simulink model "jointSpaceTrajController"  (Simulink 8.0)
settings: Solver=FixedStepDiscrete  StartTime=0.0  StopTime=10.0  FixedStep=Ts  RelTol=1e-3
libraries: WBCLibrary x5
settings Model: Creator=nunoguedelha  LastModifiedBy=nunoguedelha

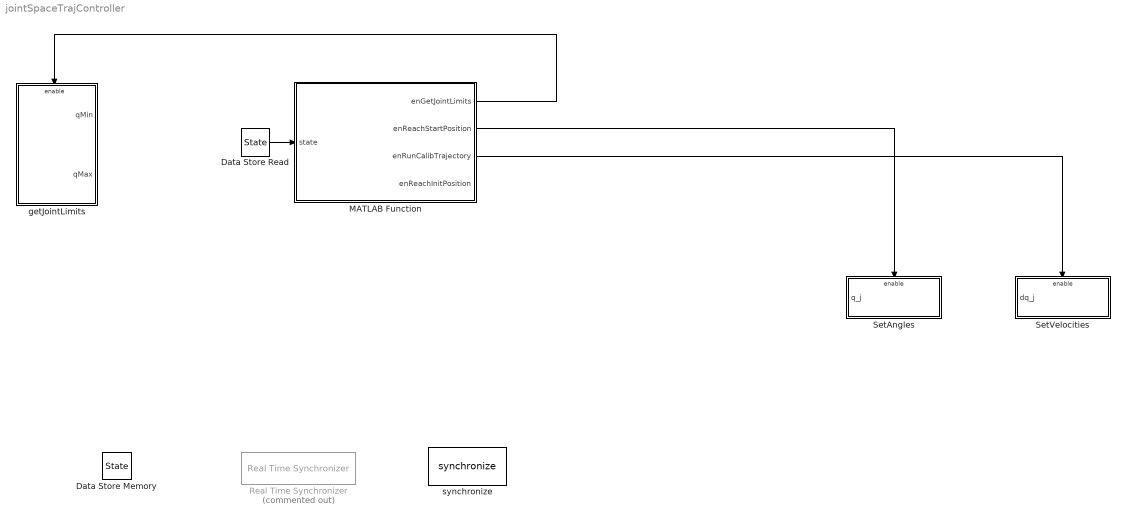
== system jointSpaceTrajController ==
  Data Store Memory : DataStoreMemory  DataStoreName=State  ReadBeforeWriteMsg=warning  WriteAfterWriteMsg=warning  WriteAfterReadMsg=warning  InitialValue=getJointLimits  OutMin=1  OutMax=4  OutDataTypeStr=Enum: SMstates
  Data Store Read : DataStoreRead  DataStoreName=State  DataStoreElements=State
  MATLAB Function : MATLAB Function  TreatAsAtomicUnit=on
  Real Time Synchronizer : WBCLibrary/Utilities/Real Time Synchronizer  Priority=-10  Commented=on  threadPeriod=Ts
  SetAngles : Subsystem  TreatAsAtomicUnit=on
  SetVelocities : Subsystem  TreatAsAtomicUnit=on
  getJointLimits : Subsystem  TreatAsAtomicUnit=on
  synchronize : WBCLibrary/Utilities/synchronize  rate=0.010  scaleFactor=1
  wires:
  MATLAB Function/2(enReachStartPosition) -> SetAngles/Enable
  MATLAB Function/3(enRunCalibTrajectory) -> SetVelocities/Enable
  MATLAB Function/1(enGetJointLimits) -> getJointLimits/Enable
  ? -> SetAngles/1(q_j)
  ? -> SetVelocities/1(dq_j)
  Data Store Read/1 -> MATLAB Function/1(state)

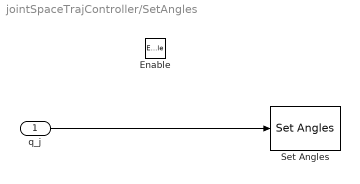
== system jointSpaceTrajController/SetAngles ==
  q_j : Inport
  Enable : EnablePort
  Set Angles : WBCLibrary/wholeBodyActuators/Set Angles  val=5  robotName=robotName  localName=localName
  wires:
  q_j/1 -> Set Angles/1

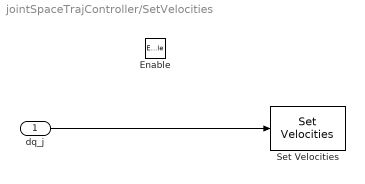
== system jointSpaceTrajController/SetVelocities ==
  dq_j : Inport
  Enable : EnablePort
  Set Velocities : WBCLibrary/wholeBodyActuators/Set Velocities  val=4  robotName=robotName  localName=localName
  wires:
  dq_j/1 -> Set Velocities/1

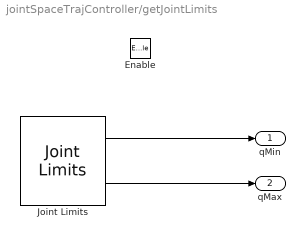
== system jointSpaceTrajController/getJointLimits ==
  Enable : EnablePort
  Joint Limits : WBCLibrary/wholeBodyModel/Joint Limits  robotName=robotName  localName=localName
  qMin : Outport
  qMax : Outport  Port=2
  wires:
  Joint Limits/1 -> qMin/1
  Joint Limits/2 -> qMax/1

== matlab function MATLAB Function ==
  data: enGetJointLimits output double; enReachStartPosition output double; enRunCalibTrajectory output double; state input double; enReachInitPosition output double
function [enGetJointLimits, enReachStartPosition, enRunCalibTrajectory, enReachInitPosition] = mainSM(state)
%#codegen

%% static variables
%

% %% States: 'getJointLimits', 'reachStartPosition', 'runCalibTrajectory'
% % 'reachInitPosition'
% persistent state;
% 
% % Init first call State
% if isempty(state)
%     state = 'getJointLimits';
% end

%% reset and set triggers from input state  
enState_getJointLimits = 0;
enReachStartPosition = 0;
enRunCalibTrajectory = 0;
enReachInitPosition = 0;

switch state
    case 1 %'getJointLimits'
        enState_getJointLimits = 1;
    case 2 %'reachStartPosition'
        enReachStartPosition = 1;
    case 3 %'runCalibTrajectory'
        enRunCalibTrajectory = 1;
    case 4 %'reachInitPosition'
        enReachInitPosition = 1;
    otherwise
        error('msgIdent','wrong state')
end
